simulink model "Full_simulink_Model"  (R2023b)
settings: Solver=VariableStepAuto  StartTime=0.0  StopTime=10.0  RelTol=1e-3
undefined symbols (not defined in the file): i_s, i_sel, J_D, Jn, Km, Kw, L_Y, Mn, R_Y
libraries: slpidlib x2
settings Model: Creator=Jadfa  LastModifiedBy=Jadfa

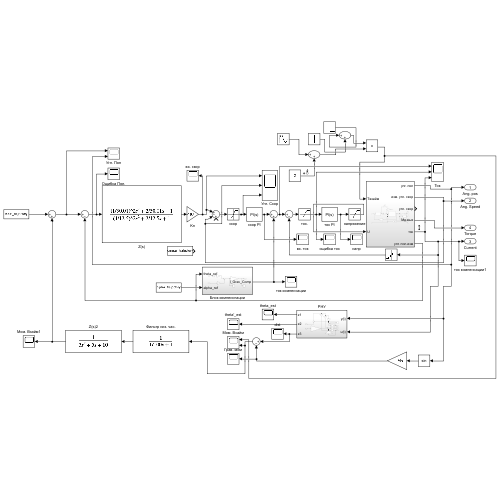
[thumbnail: Simulink's stored preview of the top-level diagram]
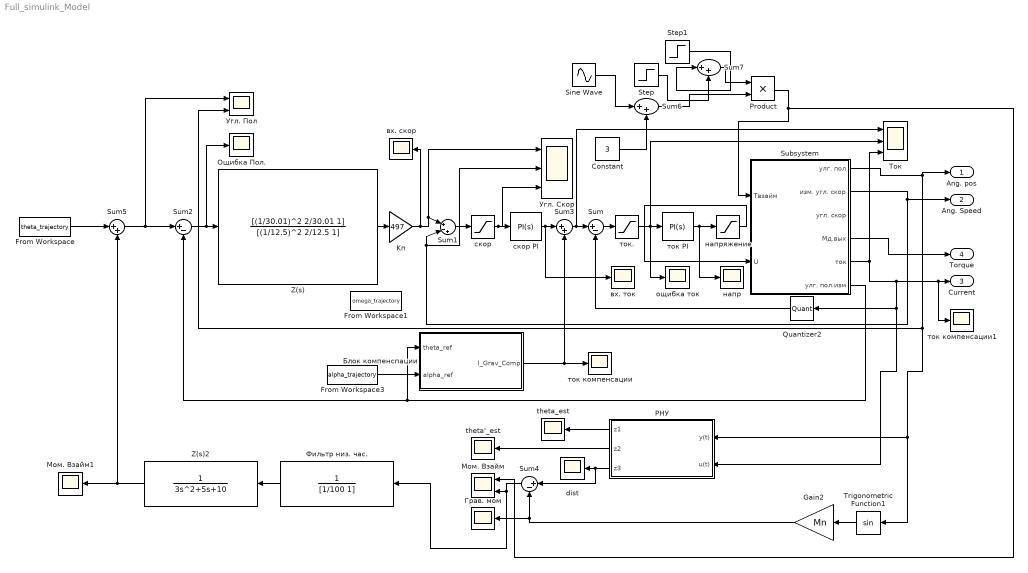
== system Full_simulink_Model ==
  Constant : Constant  Value=3
  From Workspace : FromWorkspace  VariableName=theta_trajectory
  From Workspace1 : FromWorkspace  VariableName=omega_trajectory
  From Workspace3 : FromWorkspace  VariableName=alpha_trajectory
  Gain2 : Gain  Gain=Mn
  Kп : Gain  Gain=497
  Product : Product
  Quantizer2 : Quantizer  QuantizationInterval=0.0003835
  Sine Wave : Sin  Amplitude=2  SampleTime=0
  Step : Step  Time=3  SampleTime=0
  Step1 : Step  Time=7  After=-1  SampleTime=0
  Subsystem : Subsystem
  Sum : Sum  Inputs=|+-
  Sum1 : Sum  Inputs=|+-+
  Sum2 : Sum  Inputs=|+-
  Sum{3,5..7} (4 alike) : Sum  Inputs=|++
  Sum4 : Sum  Inputs=|+-
  Trigonometric Function1 : Trigonometry
  Z(s) : TransferFcn  Numerator=[(1/30.01)^2 2/30.01 1]  Denominator=[(1/12.5)^2 2/12.5 1]
  Z(s)2 : TransferFcn  Denominator=[3 5 10]
  dist : Scope
  theta'_est : Scope
  theta_est : Scope
  Блок компенспации : Subsystem
  Грав. мом : Scope
  Мом. Взайм : Scope  NumInputPorts=2
  Мом. Взайм1 : Scope
  Ощибка Пол. : Scope
  РНУ : Subsystem
  Ток : Scope  NumInputPorts=3
  Угл. Пол : Scope  NumInputPorts=2
  Угл. Скор : Scope  NumInputPorts=3
  Фильтр низ. час. : TransferFcn  Denominator=[1/100 1]
  вх. скор : Scope
  вх. ток : Scope
  напр : Scope
  напряжение : Saturate  UpperLimit=27  LowerLimit=-27
  ощибка ток : Scope
  скор : Saturate  UpperLimit=2.09  LowerLimit=-2.09
  скор PI : slpidlib/PID Controller  Controller=PI  Form=Parallel  TimeDomain=Continuous-time  UseExternalTs=off  SampleTime=-1  IntegratorMethod=Forward Euler  FilterMethod=Forward Euler  ControllerParametersSource=internal  P=24.0169955039854  I=253.704517603607  UseKiTs=off  D=0  N=100  UseFilter=on  TunerSelectOption=Transfer Function Based (PID Tuner App)  InitialConditionSource=internal  InitialConditionForIntegrator=0  InitialConditionForFilter=0  DifferentiatorICPrevScaledInput=0  ExternalReset=none  TrackingMode=off  Kt=1  LimitOutput=off  SatLimitsSource=internal  UpperSaturationLimit=inf  LowerSaturationLimit=-inf  LinearizeAsGain=on  AntiWindupMode=none  Kb=1  LimitIntegrator=off  UpperIntegratorSaturationLimit=inf  LowerIntegratorSaturationLimit=-inf  POutMin=[]  POutMax=[]  IOutMin=[]  IOutMax=[]  DOutMin=[]  DOutMax=[]  NOutMin=[]  NOutMax=[]  SumOutMin=[]  SumOutMax=[]  SaturationOutMin=[]  SaturationOutMax=[]  PParamMin=[]  PParamMax=[]  IParamMin=[]  IParamMax=[]  DParamMin=[]  DParamMax=[]  NParamMin=[]  NParamMax=[]  KbParamMin=[]  KbParamMax=[]  KtParamMin=[]  KtParamMax=[]  KbOutMin=[]  KbOutMax=[]  KtOutMin=[]  KtOutMax=[]  IntegratorOutMin=[]  IntegratorOutMax=[]  FilterOutMin=[]  FilterOutMax=[]  SumI1OutMin=[]  SumI1OutMax=[]  SumI2OutMin=[]  SumI2OutMax=[]  SumI3OutMin=[]  SumI3OutMax=[]  SumI4OutMin=[]  SumI4OutMax=[]  SumDOutMin=[]  SumDOutMax=[]  DifferentiatorOutMin=[]  DifferentiatorOutMax=[]  FilterDiffOutCoefMin=[]  FilterDiffOutCoefMax=[]  ReciprocalOutMin=[]  ReciprocalOutMax=[]  SumDenOutMin=[]  SumDenOutMax=[]  SumNumOutMin=[]  SumNumOutMax=[]  DivideOutMin=[]  DivideOutMax=[]  UdiffTsProdOutMin=[]  UdiffTsProdOutMax=[]  NTsProdOutMin=[]  NTsProdOutMax=[]  UintegralTsProdOutMin=[]  UintegralTsProdOutMax=[]  UngainTsProdOutMin=[]  UngainTsProdOutMax=[]  ClampingZeroOutDataTypeStr=Inherit: Inherit via back propagation  ClampingZeroOutMin=[]  ClampingZeroOutMax=[]  FilterDenConstantOutDataTypeStr=Inherit: Inherit via back propagation  FilterDenConstantOutMin=[]  FilterDenConstantOutMax=[]  PCopyOutDataTypeStr=Inherit: Inherit via back propagation  PCopyOutMin=[]  PCopyOutMax=[]  NCopyOutDataTypeStr=Inherit: Inherit via back propagation  NCopyOutMin=[]  NCopyOutMax=[]  IntegratorContinuousStateAttributes=''  IntegratorStateMustResolveToSignalObject=off  IntegratorRTWStateStorageClass=Auto  FilterContinuousStateAttributes=''  FilterStateMustResolveToSignalObject=off  FilterRTWStateStorageClass=Auto  ParallelPVariant=InternalParameters  IdealPVariant=Disabled  IVariant=InternalParameters  DVariant=Disabled  IntegratorVariant=Continuous  SatVariant=Disabled  AWVariant=Passthrough  PCopyVariant=Disabled  TRVariant=Disabled  FdbkBlocksVariant=Forward  IdealPFdbkVariant=Disabled  SatFdbkVariant=Disabled  DerivativeFilterVariant=Disabled  NVariant=Disabled  NCopyVariant=Disabled_SignalSpec  FilterICVariant=Disabled  IntegratorICVariant=InternalICs  ExternalResetVariant=Disabled  TRSumVariant=Passthrough  SumFdbkVariant=Disabled  SumVariant=Sum_PI  TsampFilterVariant=InternalTs  TsampNgainVariant=Passthrough  TsampIntegralVariant=Disabled_SignalSpec  ExternalSaturationOutDataTypeStr=Inherit: Same as second input
  ток PI : slpidlib/PID Controller  Controller=PI  Form=Parallel  TimeDomain=Continuous-time  UseExternalTs=off  SampleTime=-1  IntegratorMethod=Forward Euler  FilterMethod=Forward Euler  ControllerParametersSource=internal  P=13.7877180571418  I=5650  UseKiTs=off  D=0  N=100  UseFilter=on  TunerSelectOption=Transfer Function Based (PID Tuner App)  InitialConditionSource=internal  InitialConditionForIntegrator=0  InitialConditionForFilter=0  DifferentiatorICPrevScaledInput=0  ExternalReset=none  TrackingMode=off  Kt=1  LimitOutput=off  SatLimitsSource=internal  UpperSaturationLimit=inf  LowerSaturationLimit=-inf  LinearizeAsGain=on  AntiWindupMode=none  Kb=1  LimitIntegrator=off  UpperIntegratorSaturationLimit=inf  LowerIntegratorSaturationLimit=-inf  POutMin=[]  POutMax=[]  IOutMin=[]  IOutMax=[]  DOutMin=[]  DOutMax=[]  NOutMin=[]  NOutMax=[]  SumOutMin=[]  SumOutMax=[]  SaturationOutMin=[]  SaturationOutMax=[]  PParamMin=[]  PParamMax=[]  IParamMin=[]  IParamMax=[]  DParamMin=[]  DParamMax=[]  NParamMin=[]  NParamMax=[]  KbParamMin=[]  KbParamMax=[]  KtParamMin=[]  KtParamMax=[]  KbOutMin=[]  KbOutMax=[]  KtOutMin=[]  KtOutMax=[]  IntegratorOutMin=[]  IntegratorOutMax=[]  FilterOutMin=[]  FilterOutMax=[]  SumI1OutMin=[]  SumI1OutMax=[]  SumI2OutMin=[]  SumI2OutMax=[]  SumI3OutMin=[]  SumI3OutMax=[]  SumI4OutMin=[]  SumI4OutMax=[]  SumDOutMin=[]  SumDOutMax=[]  DifferentiatorOutMin=[]  DifferentiatorOutMax=[]  FilterDiffOutCoefMin=[]  FilterDiffOutCoefMax=[]  ReciprocalOutMin=[]  ReciprocalOutMax=[]  SumDenOutMin=[]  SumDenOutMax=[]  SumNumOutMin=[]  SumNumOutMax=[]  DivideOutMin=[]  DivideOutMax=[]  UdiffTsProdOutMin=[]  UdiffTsProdOutMax=[]  NTsProdOutMin=[]  NTsProdOutMax=[]  UintegralTsProdOutMin=[]  UintegralTsProdOutMax=[]  UngainTsProdOutMin=[]  UngainTsProdOutMax=[]  ClampingZeroOutDataTypeStr=Inherit: Inherit via back propagation  ClampingZeroOutMin=[]  ClampingZeroOutMax=[]  FilterDenConstantOutDataTypeStr=Inherit: Inherit via back propagation  FilterDenConstantOutMin=[]  FilterDenConstantOutMax=[]  PCopyOutDataTypeStr=Inherit: Inherit via back propagation  PCopyOutMin=[]  PCopyOutMax=[]  NCopyOutDataTypeStr=Inherit: Inherit via back propagation  NCopyOutMin=[]  NCopyOutMax=[]  IntegratorContinuousStateAttributes=''  IntegratorStateMustResolveToSignalObject=off  IntegratorRTWStateStorageClass=Auto  FilterContinuousStateAttributes=''  FilterStateMustResolveToSignalObject=off  FilterRTWStateStorageClass=Auto  ParallelPVariant=InternalParameters  IdealPVariant=Disabled  IVariant=InternalParameters  DVariant=Disabled  IntegratorVariant=Continuous  SatVariant=Disabled  AWVariant=Passthrough  PCopyVariant=Disabled  TRVariant=Disabled  FdbkBlocksVariant=Forward  IdealPFdbkVariant=Disabled  SatFdbkVariant=Disabled  DerivativeFilterVariant=Disabled  NVariant=Disabled  NCopyVariant=Disabled_SignalSpec  FilterICVariant=Disabled  IntegratorICVariant=InternalICs  ExternalResetVariant=Disabled  TRSumVariant=Passthrough  SumFdbkVariant=Disabled  SumVariant=Sum_PI  TsampFilterVariant=InternalTs  TsampNgainVariant=Passthrough  TsampIntegralVariant=Disabled_SignalSpec  ExternalSaturationOutDataTypeStr=Inherit: Same as second input
  ток компенсации : Scope
  ток компенсации1 : Scope
  ток. : Saturate  UpperLimit=2.5  LowerLimit=-2.5
  Ang. pos : Outport
  Ang. Speed : Outport  Port=2
  Current : Outport  Port=3
  Torque : Outport  Port=4
  wires:
  From Workspace3/1 -> Блок компенспации/2(alpha_ref)
  ток PI/1 -> напряжение/1, напр/1
  Блок компенспации/1(I_Grav_Comp) -> ток компенсации/1, Sum3/2
  Z(s)/1 -> Kп/1
  Sum3/1 -> Ток/1, Sum/1
  Kп/1 -> Угл. Скор/1, Sum1/1, вх. скор/1
  РНУ/2(z2) -> theta'_est/1
  РНУ/3(z3) -> Sum4/1, dist/1
  Sum4/1 -> Фильтр низ. час./1, Мом. Взайм/2
  Subsystem/2(изм. угл. скор) -> Sum1/2, Угл. Скор/2, Ang. Speed/1
  РНУ/1(z1) -> theta_est/1
  Sum1/1 -> скор/1
  Gain2/1 -> Грав. мом/1, Sum4/2
  Subsystem/1(улг. пол) -> Ang. pos/1, Trigonometric Function1/1, РНУ/1(y(t)), Угл. Пол/2
  From Workspace/1 -> Sum5/1
  ток./1 -> ощибка ток/1, Ток/2, ток PI/1
  Subsystem/6(улг. пол.изм) -> Блок компенспации/1(theta_ref), Sum2/2
  скор PI/1 -> Sum3/1, вх. ток/1
  Sum2/1 -> Ощибка Пол./1, Z(s)/1
  скор/1 -> Угл. Скор/3, скор PI/1
  Subsystem/4(Мд.вых) -> Torque/1
  Quantizer2/1 -> Sum/2
  Subsystem/5(ток) -> РНУ/2(u(t)), Quantizer2/1, ток компенсации1/1, Current/1, Ток/3
  напряжение/1 -> Subsystem/2(U)
  Sum/1 -> ток./1
  Trigonometric Function1/1 -> Gain2/1
  Sum5/1 -> Угл. Пол/1, Sum2/1
  Product/1 -> Мом. Взайм/1, Subsystem/1(Tвзайм)
  Sum6/1 -> Product/2
  Фильтр низ. час./1 -> Z(s)2/1
  Z(s)2/1 -> Мом. Взайм1/1, Sum5/2
  Constant/1 -> Sum6/2
  Sine Wave/1 -> Sum6/1
  Step/1 -> Sum7/2
  Step1/1 -> Sum7/1
  Sum7/1 -> Product/1

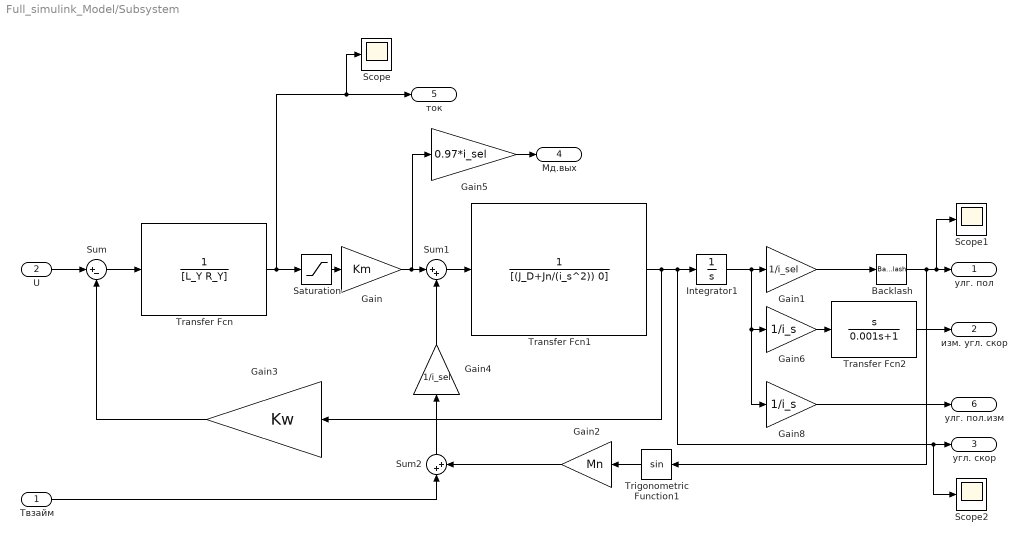
== system Full_simulink_Model/Subsystem ==
  Tвзайм : Inport
  U : Inport  Port=2
  Backlash : Backlash  BacklashWidth=0.000349
  Gain : Gain  Gain=Km
  Gain1 : Gain  Gain=1/i_sel
  Gain2 : Gain  Gain=Mn
  Gain3 : Gain  Gain=Kw
  Gain4 : Gain  Gain=1/i_sel
  Gain5 : Gain  Gain=0.97*i_sel
  Gain6 : Gain  Gain=1/i_s
  Gain8 : Gain  Gain=1/i_s
  Integrator1 : Integrator
  Saturation : Saturate  UpperLimit=6.5  LowerLimit=-6.5
  Scope : Scope
  Scope1 : Scope
  Scope2 : Scope
  Sum : Sum  Inputs=|+-
  Sum1 : Sum  Inputs=|++
  Sum2 : Sum  Inputs=|++
  Transfer Fcn : TransferFcn  Denominator=[L_Y R_Y]
  Transfer Fcn1 : TransferFcn  Denominator=[(J_D+Jn/(i_s^2)) 0]
  Transfer Fcn2 : TransferFcn  Numerator=[1 0]  Denominator=[0.001 1]
  Trigonometric Function1 : Trigonometry
  улг. пол : Outport
  изм. угл. скор : Outport  Port=2
  угл. скор : Outport  Port=3
  Мд.вых : Outport  Port=4
  ток : Outport  Port=5
  улг. пол.изм : Outport  Port=6
  wires:
  Gain3/1 -> Sum/2
  U/1 -> Sum/1
  Transfer Fcn1/1 -> Integrator1/1, Scope2/1, угл. скор/1, Gain3/1
  Sum1/1 -> Transfer Fcn1/1
  Sum/1 -> Transfer Fcn/1
  Transfer Fcn/1 -> Scope/1, ток/1, Saturation/1
  Trigonometric Function1/1 -> Gain2/1
  Transfer Fcn2/1 -> изм. угл. скор/1
  Gain5/1 -> Мд.вых/1
  Gain/1 -> Gain5/1, Sum1/1
  Saturation/1 -> Gain/1
  Sum2/1 -> Gain4/1
  Integrator1/1 -> Gain8/1, Gain6/1, Gain1/1
  Tвзайм/1 -> Sum2/1
  Backlash/1 -> Trigonometric Function1/1, Scope1/1, улг. пол/1
  Gain1/1 -> Backlash/1
  Gain6/1 -> Transfer Fcn2/1
  Gain8/1 -> улг. пол.изм/1
  Gain2/1 -> Sum2/2
  Gain4/1 -> Sum1/2

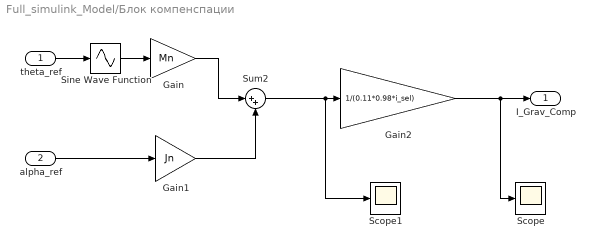
== system Full_simulink_Model/Блок компенспации ==
  theta_ref : Inport
  alpha_ref : Inport  Port=2
  Gain : Gain  Gain=Mn
  Gain1 : Gain  Gain=Jn
  Gain2 : Gain  Gain=1/(0.11*0.98*i_sel)
  Scope : Scope
  Scope1 : Scope
  Sine Wave Function : Sin  TimeSource=Use external signal  SampleTime=0
  Sum2 : Sum  Inputs=|++
  I_Grav_Comp : Outport
  wires:
  Gain/1 -> Sum2/1
  alpha_ref/1 -> Gain1/1
  Sum2/1 -> Scope1/1, Gain2/1
  Sine Wave Function/1 -> Gain/1
  theta_ref/1 -> Sine Wave Function/1
  Gain2/1 -> Scope/1, I_Grav_Comp/1
  Gain1/1 -> Sum2/2

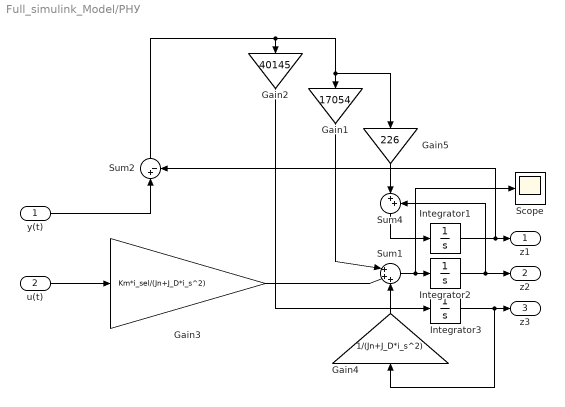
== system Full_simulink_Model/РНУ ==
  y(t) : Inport
  u(t) : Inport  Port=2
  Gain1 : Gain  Gain=17054
  Gain2 : Gain  Gain=40145
  Gain3 : Gain  Gain=Km*i_sel/(Jn+J_D*i_s^2)
  Gain4 : Gain  Gain=1/(Jn+J_D*i_s^2)
  Gain5 : Gain  Gain=226
  Integrator1 : Integrator
  Integrator2 : Integrator
  Integrator3 : Integrator
  Scope : Scope
  Sum1 : Sum  Inputs=|+++
  Sum2 : Sum  Inputs=|+-
  Sum4 : Sum  Inputs=|++
  z1 : Outport
  z2 : Outport  Port=2
  z3 : Outport  Port=3
  wires:
  u(t)/1 -> Gain3/1
  Integrator1/1 -> z1/1, Sum2/2
  y(t)/1 -> Sum2/1
  Sum2/1 -> Gain5/1, Gain1/1, Gain2/1
  Gain2/1 -> Integrator3/1
  Sum1/1 -> Scope/1, Integrator2/1
  Gain4/1 -> Sum1/3
  Gain3/1 -> Sum1/2
  Gain1/1 -> Sum1/1
  Gain5/1 -> Sum4/1
  Sum4/1 -> Integrator1/1
  Integrator2/1 -> Sum4/2, z2/1
  Integrator3/1 -> Gain4/1, z3/1
